simulink model "mars_rover_pose"  (R2023a)
settings: Solver=ode23t  StartTime=0.0  StopTime=2000  FixedStep=1e-2  MaxStep=0.1  RelTol=1e-3  AbsTol=1e-3  EnableMultiTasking=on
StartFcn:
  | mars_rover_sim_callback
model workspace (MATLAB code in the model file):
  | addpath("mars_rover_helpers");
  | % Load Rover Arm model for IK
  | mdlpath = ['mars_rover_data',filesep,'mars_rover_arm'];
  | load_system(mdlpath);
  | 
  | imdata = zeros(3,3,3);
  | 
  | % Temp
  | Kp_steer = 1;
  | Ki_steer = 1;
  | Kd_steer = 1;
  | 
  | Kp = 1;
  | Ki = 1;
  | Kd = 1;
values from neighbouring files (symbols this model uses):
  mapData = false(197,200)    [mars_rover_params.m]    (also in mars_rover_startup.m)
  useKalmanFilter = true    [mars_rover_params.m]
undefined symbols (not defined in the file or in its folder): Arm, armJointAng, armJointTrqs, cameraData, eeConfig, pose, Rover, rover_path_dl, roverPath, sampleLocation, steerAng, steerTrqs, Terrain, vSpeed, Wheel1_G, Wheel2_G, Wheel3_G, Wheel4_G, Wheel5_G, Wheel6_G, wheelTrqs, wSpeeds, X, Y, Z
libraries: sm_lib x238, nesl_utility x80, slpidlib x3, simulink x3, robotcorelib x2, simulink_extras x2, robotalgslib x1
(part 8 of 9)

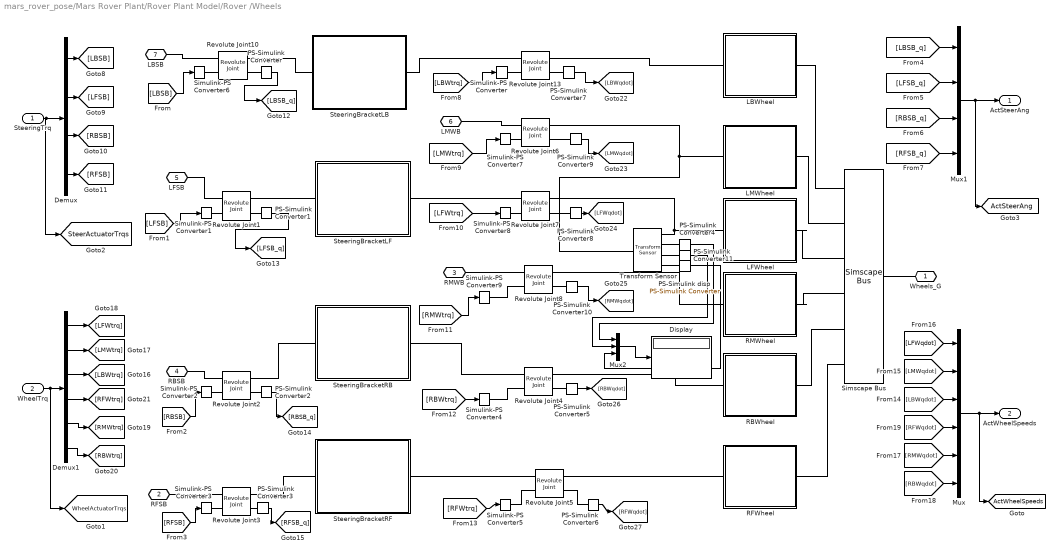
== system mars_rover_pose/Mars Rover Plant/Rover Plant Model/Rover /Wheels ==
  SteeringTrq : Inport
  WheelTrq : Inport  Port=2
  Demux : Demux
  Demux1 : Demux  Outputs=6
  Display : Display
  LBWheel : Subsystem
  LFWheel : Subsystem
  LMWheel : Subsystem
  Mux : Mux  Inputs=6
  Mux1 : Mux
  Mux2 : Mux  Inputs=3
  PS-Simulink Converter{,1..3} (4 alike) : nesl_utility/PS-Simulink Converter  PhysicalDomain=network_engine_domain  SubClassName=ps_output  LeftPortType=input  RightPortType=output  PseudoPeriodic=off  Frequencies=[]  VectorFormat=1-D array  Unit=deg  AffineConversion=off
  PS-Simulink Converter{5..10} (6 alike) : nesl_utility/PS-Simulink Converter  PhysicalDomain=network_engine_domain  SubClassName=ps_output  LeftPortType=input  RightPortType=output  PseudoPeriodic=off  Frequencies=[]  VectorFormat=1-D array  Unit=inherit  AffineConversion=off
  PS-Simulink Converter11 : nesl_utility/PS-Simulink Converter  PhysicalDomain=network_engine_domain  SubClassName=ps_output  LeftPortType=input  RightPortType=output  PseudoPeriodic=off  Frequencies=[]  VectorFormat=inherit  Unit=inherit  AffineConversion=off
  PS-Simulink Converter4 : nesl_utility/PS-Simulink Converter  PhysicalDomain=network_engine_domain  SubClassName=ps_output  LeftPortType=input  RightPortType=output  PseudoPeriodic=off  Frequencies=[]  VectorFormat=inherit  Unit=inherit  AffineConversion=off
  PS-Simulink disp : nesl_utility/PS-Simulink Converter  PhysicalDomain=network_engine_domain  SubClassName=ps_output  LeftPortType=input  RightPortType=output  PseudoPeriodic=off  Frequencies=[]  VectorFormat=inherit  Unit=inherit  AffineConversion=off
  RBWheel : Subsystem
  RFWheel : Subsystem
  RMWheel : Subsystem
  Revolute Joint{1..3,10} (4 alike) : sm_lib/Joints/Revolute Joint  JointMode=Normal  SenseConstraintForce=off  SenseConstraintForceX=off  SenseConstraintForceY=off  SenseConstraintForceZ=off  SenseConstraintTorque=off  SenseConstraintTorqueX=off  SenseConstraintTorqueY=off  SenseConstraintTorqueZ=off  SenseTotalForce=off  SenseTotalForceX=off  SenseTotalForceY=off  SenseTotalForceZ=off  SenseTotalTorque=off  SenseTotalTorqueX=off  SenseTotalTorqueY=off  SenseTotalTorqueZ=off  CompositeWrenchDir=FollowerOnBase  CompositeWrenchFrame=BaseFrame  EquilibriumPosition=0  EquilibriumPositionUnits=deg  SpringStiffness=0  SpringStiffnessUnits=N*m/deg  DampingCoefficient=Rover.steering_damping  DampingCoefficientUnits=N*m/(deg/s)  TorqueActuationMode=InputTorque  MotionActuationMode=ComputedMotion  SensePosition=on  SenseVelocity=off  SenseAcceleration=off  SenseTorqueForce=off  SenseLowerLimitTorqueForce=off  SenseUpperLimitTorqueForce=off  LowerLimitSpecify=off  LowerLimitBound=-90  LowerLimitBoundUnits=deg  LowerLimitStiffness=1e4  LowerLimitStiffnessUnits=N*m/deg  LowerLimitDamping=10  LowerLimitDampingUnits=N*m/(deg/s)  LowerLimitTransitionRegionWidth=0.1  LowerLimitTransitionRegionWidthUnits=deg  UpperLimitSpecify=off  UpperLimitBound=90  UpperLimitBoundUnits=deg  UpperLimitStiffness=1e4  UpperLimitStiffnessUnits=N*m/deg  UpperLimitDamping=10  UpperLimitDampingUnits=N*m/(deg/s)  UpperLimitTransitionRegionWidth=0.1  UpperLimitTransitionRegionWidthUnits=deg  PositionTargetSpecify=on  PositionTargetPriority=High  PositionTargetValue=0  PositionTargetValueUnits=deg  VelocityTargetSpecify=off  VelocityTargetPriority=High  VelocityTargetValue=0  VelocityTargetValueUnits=deg/s
  Revolute Joint{4..8,13} (6 alike) : sm_lib/Joints/Revolute Joint  JointMode=Normal  SenseConstraintForce=off  SenseConstraintForceX=off  SenseConstraintForceY=off  SenseConstraintForceZ=off  SenseConstraintTorque=off  SenseConstraintTorqueX=off  SenseConstraintTorqueY=off  SenseConstraintTorqueZ=off  SenseTotalForce=off  SenseTotalForceX=off  SenseTotalForceY=off  SenseTotalForceZ=off  SenseTotalTorque=off  SenseTotalTorqueX=off  SenseTotalTorqueY=off  SenseTotalTorqueZ=off  CompositeWrenchDir=FollowerOnBase  CompositeWrenchFrame=BaseFrame  EquilibriumPosition=0  EquilibriumPositionUnits=deg  SpringStiffness=0  SpringStiffnessUnits=N*m/deg  DampingCoefficient=Rover.wheel_damping  DampingCoefficientUnits=N*m/(deg/s)  TorqueActuationMode=InputTorque  MotionActuationMode=ComputedMotion  SensePosition=off  SenseVelocity=on  SenseAcceleration=off  SenseTorqueForce=off  SenseLowerLimitTorqueForce=off  SenseUpperLimitTorqueForce=off  LowerLimitSpecify=off  LowerLimitBound=-90  LowerLimitBoundUnits=deg  LowerLimitStiffness=1e4  LowerLimitStiffnessUnits=N*m/deg  LowerLimitDamping=10  LowerLimitDampingUnits=N*m/(deg/s)  LowerLimitTransitionRegionWidth=0.1  LowerLimitTransitionRegionWidthUnits=deg  UpperLimitSpecify=off  UpperLimitBound=90  UpperLimitBoundUnits=deg  UpperLimitStiffness=1e4  UpperLimitStiffnessUnits=N*m/deg  UpperLimitDamping=10  UpperLimitDampingUnits=N*m/(deg/s)  UpperLimitTransitionRegionWidth=0.1  UpperLimitTransitionRegionWidthUnits=deg  PositionTargetSpecify=off  PositionTargetPriority=High  PositionTargetValue=0  PositionTargetValueUnits=deg  VelocityTargetSpecify=off  VelocityTargetPriority=High  VelocityTargetValue=0  VelocityTargetValueUnits=deg/s
  Simscape Bus : SimscapeBus  HierarchyStrings=Wheel1_G;Wheel2_G;Wheel3_G;Wheel4_G;Wheel5_G;Wheel6_G
  Simulink-PS Converter{,4..5,7..9} (6 alike) : nesl_utility/Simulink-PS Converter  PhysicalDomain=network_engine_domain  SubClassName=ps_input  LeftPortType=input  RightPortType=output  PseudoPeriodic=off  Frequencies=[]  NoiseDistribution=none  NoiseParameters=[]  Unit=1  AffineConversion=off  FilteringAndDerivatives=provide  SimscapeFilterOrder=1  InputFilterTimeConstant=0.001  UdotUserProvided=0
  Simulink-PS Converter{1..3,6} (4 alike) : nesl_utility/Simulink-PS Converter  PhysicalDomain=network_engine_domain  SubClassName=ps_input  LeftPortType=input  RightPortType=output  PseudoPeriodic=off  Frequencies=[]  NoiseDistribution=none  NoiseParameters=[]  Unit=1  AffineConversion=off  FilteringAndDerivatives=zero  SimscapeFilterOrder=2  InputFilterTimeConstant=0.001  UdotUserProvided=0
  "SteeringBracketLB " : Subsystem
  SteeringBracketLF : Subsystem
  SteeringBracketRB : Subsystem
  SteeringBracketRF : Subsystem
  Transform Sensor : sm_lib/Frames and Transforms/Transform Sensor  MeasurementFrame=Base  RotationSequence=XYX  SenseAngle=off  SenseAxis=off  SenseQ=off  SenseR=off  SenseRotationSequence=off  SenseOmegaX=off  SenseOmegaY=off  SenseOmegaZ=off  SenseQDot=off  SenseRDot=off  SenseRotationSequenceDot=off  SenseAlphaX=off  SenseAlphaY=off  SenseAlphaZ=off  SenseQDDot=off  SenseRDDot=off  SenseX=on  SenseY=on  SenseZ=on  SenseRad=off  SenseAzim=off  SenseDist=off  SenseInc=off  SenseXDot=off  SenseYDot=off  SenseZDot=off  SenseRadDot=off  SenseAzimDot=off  SenseDistDot=off  SenseIncDot=off  SenseXDDot=off  SenseYDDot=off  SenseZDDot=off  SenseRadDDot=off  SenseAzimDDot=off  SenseDistDDot=off  SenseIncDDot=off
  Wheels_G : PMIOPort  Side=Left
  RFSB : PMIOPort  Port=2  Side=Left
  RMWB : PMIOPort  Port=3  Side=Left
  RBSB : PMIOPort  Port=4  Side=Left
  LFSB : PMIOPort  Port=5  Side=Right
  LMWB : PMIOPort  Port=6  Side=Right
  LBSB : PMIOPort  Port=7  Side=Right
  ActSteerAng : Outport
  ActWheelSpeeds : Outport  Port=2
  tag scope: ActSteerAng=global, ActWheelSpeeds=global, SteerActuatorTrqs=global, WheelActuatorTrqs=global
  wires:
  SteeringTrq/1 -> [SteerActuatorTrqs], Demux/1
  Mux1/1 -> ActSteerAng/1, [ActSteerAng]
  WheelTrq/1 -> Demux1/1, [WheelActuatorTrqs]
  [LBSB] -> Simulink-PS Converter6/1
  Demux/1 -> [LBSB]
  Demux/2 -> [LFSB]
  Demux/3 -> [RBSB]
  Demux/4 -> [RFSB]
  [LFSB] -> Simulink-PS Converter1/1
  [RBSB] -> Simulink-PS Converter2/1
  [RFSB] -> Simulink-PS Converter3/1
  [LBSB_q] -> Mux1/1
  [LFSB_q] -> Mux1/2
  [RBSB_q] -> Mux1/3
  [RFSB_q] -> Mux1/4
  PS-Simulink Converter/1 -> [LBSB_q]
  PS-Simulink Converter1/1 -> [LFSB_q]
  PS-Simulink Converter2/1 -> [RBSB_q]
  PS-Simulink Converter3/1 -> [RFSB_q]
  [LBWtrq] -> Simulink-PS Converter/1
  [LMWtrq] -> Simulink-PS Converter7/1
  Demux1/3 -> [LBWtrq]
  Demux1/2 -> [LMWtrq]
  [LFWtrq] -> Simulink-PS Converter8/1
  Demux1/1 -> [LFWtrq]
  [RMWtrq] -> Simulink-PS Converter9/1
  Demux1/5 -> [RMWtrq]
  [RBWtrq] -> Simulink-PS Converter4/1
  Demux1/6 -> [RBWtrq]
  [RFWtrq] -> Simulink-PS Converter5/1
  Demux1/4 -> [RFWtrq]
  PS-Simulink Converter7/1 -> [LBWqdot]
  [LBWqdot] -> Mux/3
  PS-Simulink Converter9/1 -> [LMWqdot]
  [LMWqdot] -> Mux/2
  PS-Simulink Converter8/1 -> [LFWqdot]
  [LFWqdot] -> Mux/1
  PS-Simulink Converter10/1 -> [RMWqdot]
  PS-Simulink Converter5/1 -> [RBWqdot]
  PS-Simulink Converter6/1 -> [RFWqdot]
  [RMWqdot] -> Mux/5
  [RBWqdot] -> Mux/6
  [RFWqdot] -> Mux/4
  Mux/1 -> ActWheelSpeeds/1, [ActWheelSpeeds]
  Mux2/1 -> Display/1
  PS-Simulink Converter4/1 -> Mux2/1
  PS-Simulink Converter11/1 -> Mux2/2
  PS-Simulink disp/1 -> Mux2/3
  connections:
  PS-Simulink Converter/LConn1 -- Revolute Joint10/RConn2
  Revolute Joint10/LConn1 -- LBSB/RConn1
  Simulink-PS Converter6/RConn1 -- Revolute Joint10/LConn2
  "SteeringBracketLB "/LConn1 -- Revolute Joint10/RConn1
  Revolute Joint6/LConn1 -- LMWB/RConn1
  LFSB/RConn1 -- Revolute Joint1/LConn1
  Revolute Joint8/LConn1 -- RMWB/RConn1
  RBSB/RConn1 -- Revolute Joint2/LConn1
  PS-Simulink Converter1/LConn1 -- Revolute Joint1/RConn2
  Simulink-PS Converter1/RConn1 -- Revolute Joint1/LConn2
  Revolute Joint2/RConn1 -- SteeringBracketRB/LConn1
  PS-Simulink Converter2/LConn1 -- Revolute Joint2/RConn2
  Simulink-PS Converter2/RConn1 -- Revolute Joint2/LConn2
  RFSB/RConn1 -- Revolute Joint3/LConn1
  Revolute Joint3/RConn1 -- SteeringBracketRF/LConn1
  Simulink-PS Converter3/RConn1 -- Revolute Joint3/LConn2
  PS-Simulink Converter3/LConn1 -- Revolute Joint3/RConn2
  Wheels_G/RConn1 -- Simscape Bus/RConn1
  LMWheel/LConn1 -- Simscape Bus/LConn2
  RMWheel/LConn1 -- Simscape Bus/LConn4
  LFWheel/LConn1 -- Simscape Bus/LConn3
  Revolute Joint4/LConn1 -- SteeringBracketRB/RConn1
  Revolute Joint1/RConn1 -- SteeringBracketLF/LConn1
  Revolute Joint4/RConn1 -- RBWheel/RConn1
  LBWheel/RConn1 -- Revolute Joint13/RConn1
  LMWheel/RConn1 -- Revolute Joint6/RConn1 -- Transform Sensor/LConn1
  PS-Simulink Converter6/LConn1 -- Revolute Joint5/RConn2
  Revolute Joint8/LConn2 -- Simulink-PS Converter9/RConn1
  Revolute Joint13/LConn1 -- "SteeringBracketLB "/RConn1
  Simscape Bus/LConn5 -- RBWheel/LConn1
  Simulink-PS Converter5/RConn1 -- Revolute Joint5/LConn2
  Revolute Joint4/RConn2 -- PS-Simulink Converter5/LConn1
  Revolute Joint8/RConn2 -- PS-Simulink Converter10/LConn1
  Revolute Joint4/LConn2 -- Simulink-PS Converter4/RConn1
  Revolute Joint5/LConn1 -- SteeringBracketRF/RConn1
  Revolute Joint6/LConn2 -- Simulink-PS Converter7/RConn1
  Revolute Joint6/RConn2 -- PS-Simulink Converter9/LConn1
  Simscape Bus/LConn1 -- LBWheel/LConn1
  Revolute Joint13/RConn2 -- PS-Simulink Converter7/LConn1
  Revolute Joint7/LConn2 -- Simulink-PS Converter8/RConn1
  Revolute Joint7/RConn2 -- PS-Simulink Converter8/LConn1
  RMWheel/RConn1 -- Revolute Joint8/RConn1
  Revolute Joint7/LConn1 -- SteeringBracketLF/RConn1
  Simulink-PS Converter/RConn1 -- Revolute Joint13/LConn2
  LFWheel/RConn1 -- Revolute Joint7/RConn1 -- Transform Sensor/RConn1
  RFWheel/LConn1 -- Simscape Bus/LConn6
  Revolute Joint5/RConn1 -- RFWheel/RConn1
  PS-Simulink Converter4/LConn1 -- Transform Sensor/RConn2
  PS-Simulink Converter11/LConn1 -- Transform Sensor/RConn3
  PS-Simulink disp/LConn1 -- Transform Sensor/RConn4

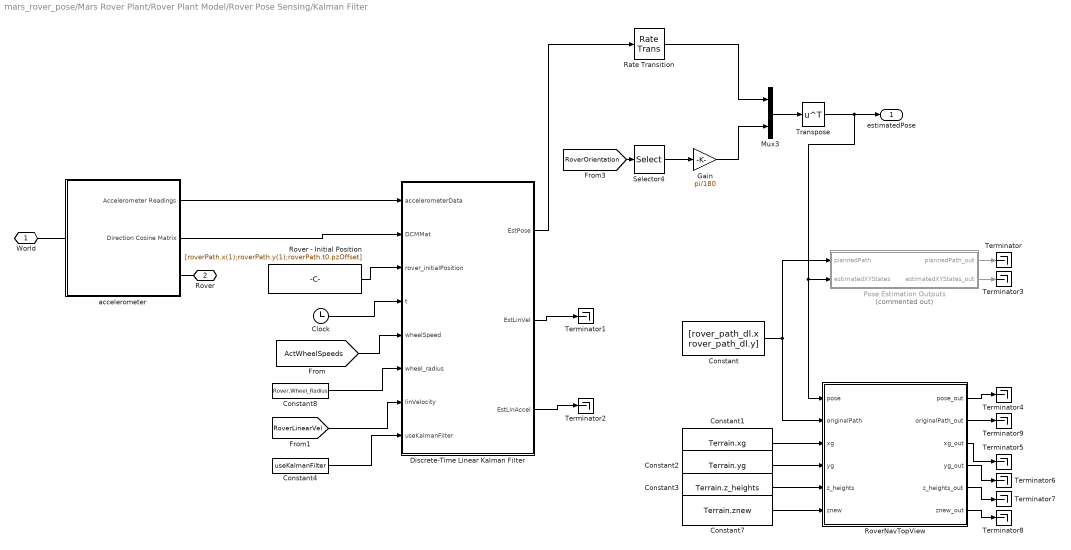
== system mars_rover_pose/Mars Rover Plant/Rover Plant Model/Rover Pose Sensing/Kalman Filter ==
  Clock : Clock
  Constant : Constant  Value=[rover_path_dl.x rover_path_dl.y]
  Constant1 : Constant  Value=Terrain.xg
  Constant2 : Constant  Value=Terrain.yg
  Constant3 : Constant  Value=Terrain.z_heights
  Constant4 : Constant  Value=useKalmanFilter
  Constant7 : Constant  Value=Terrain.znew
  Constant8 : Constant  Value=Rover.Wheel_Radius
  Discrete-Time Linear Kalman Filter : MATLAB Function  TreatAsAtomicUnit=on
  Gain : Gain  Gain=pi/180
  Mux3 : Mux  Inputs=2
  Pose Estimation Outputs : MATLAB Function  Commented=on  TreatAsAtomicUnit=on
  Rate Transition : RateTransition  InitialCondition=[roverPath.x(1) roverPath.y(1)]  OutPortSampleTime=10
  Rover - Initial Position : Constant  Value=[roverPath.x(1);roverPath.y(1);roverPath.t0.pzOffset]
  RoverNavTopView : MATLAB Function  TreatAsAtomicUnit=on
  Selector4 : Selector  InputPortWidth=3  IndexOptions=Index vector (dialog)  Indices=3  OutputSizes=1
  Terminator{,1..9} (10 alike) : Terminator
  Transpose : Math  Operator=transpose
  accelerometer : Subsystem
  World : PMIOPort  Side=Left
  Rover : PMIOPort  Port=2  Side=Right
  estimatedPose : Outport
  wires:
  Discrete-Time Linear Kalman Filter/2(EstLinVel) -> Terminator1/1
  Selector4/1 -> Gain/1
  accelerometer/2(Direction Cosine Matrix) -> Discrete-Time Linear Kalman Filter/2(DCMMat)
  [RoverOrientation] -> Selector4/1
  Discrete-Time Linear Kalman Filter/3(EstLinAccel) -> Terminator2/1
  accelerometer/1(Accelerometer Readings) -> Discrete-Time Linear Kalman Filter/1(accelerometerData)
  Constant8/1 -> Discrete-Time Linear Kalman Filter/6(wheel_radius)
  Rover - Initial Position/1 -> Discrete-Time Linear Kalman Filter/3(rover_initialPosition)
  Transpose/1 -> RoverNavTopView/1(pose), Pose Estimation Outputs/2(estimatedXYStates), estimatedPose/1
  Discrete-Time Linear Kalman Filter/1(EstPose) -> Rate Transition/1
  Mux3/1 -> Transpose/1
  Gain/1 -> Mux3/2
  Rate Transition/1 -> Mux3/1
  [ActWheelSpeeds] -> Discrete-Time Linear Kalman Filter/5(wheelSpeed)
  Clock/1 -> Discrete-Time Linear Kalman Filter/4(t)
  [RoverLinearVel] -> Discrete-Time Linear Kalman Filter/7(linVelocity)
  Pose Estimation Outputs/1(plannedPath_out) -> Terminator/1
  Pose Estimation Outputs/2(estimatedXYStates_out) -> Terminator3/1
  Constant/1 -> RoverNavTopView/2(originalPath), Pose Estimation Outputs/1(plannedPath)
  Constant3/1 -> RoverNavTopView/5(z_heights)
  Constant2/1 -> RoverNavTopView/4(yg)
  Constant1/1 -> RoverNavTopView/3(xg)
  RoverNavTopView/3(xg_out) -> Terminator5/1
  Constant7/1 -> RoverNavTopView/6(znew)
  RoverNavTopView/5(z_heights_out) -> Terminator7/1
  RoverNavTopView/4(yg_out) -> Terminator6/1
  RoverNavTopView/6(znew_out) -> Terminator8/1
  RoverNavTopView/1(pose_out) -> Terminator4/1
  RoverNavTopView/2(originalPath_out) -> Terminator9/1
  Constant4/1 -> Discrete-Time Linear Kalman Filter/8(useKalmanFilter)
  connections:
  accelerometer/LConn1 -- World/RConn1
  accelerometer/RConn1 -- Rover/RConn1

== system mars_rover_pose/Mars Rover Plant/Rover Plant Model/Rover Pose Sensing/Subsystem ==
  posX : Inport
  vx : Inport  Port=2
  posY : Inport  Port=3
  vy : Inport  Port=4
  posZ : Inport  Port=5
  Q : Inport  Port=6
  CalcSpeed : MATLAB Function  TreatAsAtomicUnit=on
  Mux : Mux  Inputs=3
  Mux1 : Mux  Inputs=2
  Mux2 : Mux  Inputs=3
  Mux3 : Mux  Inputs=3
  Radians to Degrees : simulink_extras/Transformations/Radians to Degrees
  theta_act : MATLAB Function  TreatAsAtomicUnit=on
  pose : Outport
  xyz : Outport  Port=2
  linVelxy : Outport  Port=3
  vSpeed : Outport  Port=4
  rotang : Outport  Port=5
  wires:
  posY/1 -> Mux/2, Mux3/2
  Mux1/1 -> linVelxy/1, CalcSpeed/1(u)
  Mux2/1 -> Radians to Degrees/1
  theta_act/1(z) -> Mux2/3, Mux/3
  Radians to Degrees/1 -> rotang/1
  theta_act/3(x) -> Mux2/1
  theta_act/2(y) -> Mux2/2
  posX/1 -> Mux3/1, Mux/1
  vx/1 -> Mux1/1
  Mux/1 -> pose/1
  Q/1 -> theta_act/1(u)
  vy/1 -> Mux1/2
  posZ/1 -> Mux3/3
  CalcSpeed/1(y) -> vSpeed/1
  Mux3/1 -> xyz/1

== system mars_rover_pose/Perception/sceneViewer/Stereo_Left/drawScene ==
  Camera_Z_ang : Inport
  Camera_pos : Inport  Port=2
  Camera_rot : Inport  Port=3
  Camera_target_ang : Inport  Port=4
  xg : Inport  Port=5
  yg : Inport  Port=6
  z_heights : Inport  Port=7
  znew : Inport  Port=8
  rover_path_x : Inport  Port=9
  rover_path_y : Inport  Port=10
  rover_path_z : Inport  Port=11
  Trigger : TriggerPort  VariantControl=(inherit)  InitialTriggerSignalState=negative  PortDimensions=1
  Camera : MATLAB Function  TreatAsAtomicUnit=on
  im : Outport
  wires:
  Camera/1(im) -> im/1
  rover_path_x/1 -> Camera/9(rover_path_x)
  Camera_Z_ang/1 -> Camera/1(Camera_Z_ang)
  rover_path_z/1 -> Camera/11(rover_path_z)
  z_heights/1 -> Camera/7(z_heights)
  xg/1 -> Camera/5(xg)
  znew/1 -> Camera/8(znew)
  rover_path_y/1 -> Camera/10(rover_path_y)
  yg/1 -> Camera/6(yg)
  Camera_pos/1 -> Camera/2(Camera_pos)
  Camera_target_ang/1 -> Camera/4(Camera_target_ang)
  Camera_rot/1 -> Camera/3(Camera_rot)

== system mars_rover_pose/Perception/sceneViewer/Stereo_Right/drawScene ==
  Camera_Z_ang : Inport
  Camera_pos : Inport  Port=2
  Camera_rot : Inport  Port=3
  Camera_target_ang : Inport  Port=4
  xg : Inport  Port=5
  yg : Inport  Port=6
  z_heights : Inport  Port=7
  znew : Inport  Port=8
  rover_path_x : Inport  Port=9
  rover_path_y : Inport  Port=10
  rover_path_z : Inport  Port=11
  Trigger : TriggerPort  VariantControl=(inherit)  InitialTriggerSignalState=negative  PortDimensions=1
  Camera : MATLAB Function  TreatAsAtomicUnit=on
  im : Outport
  wires:
  Camera/1(im) -> im/1
  Camera_pos/1 -> Camera/2(Camera_pos)
  rover_path_z/1 -> Camera/11(rover_path_z)
  Camera_target_ang/1 -> Camera/4(Camera_target_ang)
  rover_path_y/1 -> Camera/10(rover_path_y)
  znew/1 -> Camera/8(znew)
  z_heights/1 -> Camera/7(z_heights)
  xg/1 -> Camera/5(xg)
  rover_path_x/1 -> Camera/9(rover_path_x)
  yg/1 -> Camera/6(yg)
  Camera_Z_ang/1 -> Camera/1(Camera_Z_ang)
  Camera_rot/1 -> Camera/3(Camera_rot)

== system mars_rover_pose/Control/Manipulator Control/ Trajectory Planner/SampleDropOffCmdLogic/Enabled Subsystem1 ==
  In1 : Inport
  Enable : EnablePort
  Out1 : Outport
  wires:
  In1/1 -> Out1/1

== system mars_rover_pose/Control/Manipulator Control/ Trajectory Planner/SampleLoc wrt arm base/Enabled Subsystem1 ==
  In1 : Inport
  Enable : EnablePort
  Out1 : Outport
  wires:
  In1/1 -> Out1/1

== system mars_rover_pose/Control/Manipulator Control/ Trajectory Planner/SamplePickUpCmdLogic/Enabled Subsystem1 ==
  In1 : Inport
  Enable : EnablePort
  Out1 : Outport
  wires:
  In1/1 -> Out1/1

== system mars_rover_pose/Control/Rover Control/Rover Path Planning And Control/Ackerman Steer Angle/Enabled Subsystem ==
  In1 : Inport
  Enable : EnablePort
  delta : Outport
  wires:
  In1/1 -> delta/1

== system mars_rover_pose/Control/Rover Control/Rover Path Planning And Control/hold/RoverStopTime ==
  Enable : Inport
  Clock : Clock
  Constant2 : Constant
  Display : Display
  Enabled Subsystem1 : Subsystem  TreatAsAtomicUnit=on
      settings: MinAlgLoopOccurrences=on
  Switch : Switch  Criteria=u2 > Threshold  SaturateOnIntegerOverflow=off  InputSameDT=off
  Unit Delay : UnitDelay  SampleTime=-1  HasFrameUpgradeWarning=on
  DeAccelTime : Outport
  wires:
  Enabled Subsystem1/1(Out1) -> Switch/2
  Enable/1 -> Enabled Subsystem1/Enable
  Switch/1 -> Unit Delay/1
  Unit Delay/1 -> Display/1, DeAccelTime/1, Switch/1
  Clock/1 -> Switch/3
  Constant2/1 -> Enabled Subsystem1/1(In1)

== system mars_rover_pose/Mars Rover Plant/Manipulator Plant Model/SampleGeneration/SampleLoc wrt arm base/Enabled Subsystem1 ==
  In1 : Inport
  Enable : EnablePort
  Out1 : Outport
  wires:
  In1/1 -> Out1/1

== system mars_rover_pose/Mars Rover Plant/Rover Plant Model/Rover /Wheels/LBWheel ==
  InnerWheelViz : sm_lib/Body Elements/File Solid  ExtGeomFileName=mobility_wheel_inner.stl  UnitType=Custom  ExtGeomFileUnits=cm  StepReaderType=HEX  ExportConvexHullGeometry=off  InertiaType=Custom  Mass=0  MassUnits=kg  CenterOfMass=[0 0 0]  CenterOfMassUnits=m  MomentsOfInertia=[1 1 1]*0  MomentsOfInertiaUnits=kg*m^2  ProductsOfInertia=[0 0 0]  ProductsOfInertiaUnits=kg*m^2  BasedOnType=Density  Density=1000  DensityUnits=kg/m^3  DoExposeReferenceFrame=on  SerializedFrames=<Frames/>  GraphicType=FromGeometry  MarkerShape=Sphere  MarkerSize=10  GraphicVisPropType=AdvancedVisualProperties  GraphicDiffuseColor=[1.0 1.0 1.0]  GraphicSpecularColor=[1 1 1 1.0]  GraphicAmbientColor=[0.15 0.15 0.15 1.0]  GraphicEmissiveColor=[0.1 0.1 0 1.0]  GraphicShininess=90  GraphicOpacity=1.0
  OuterWheel : sm_lib/Body Elements/File Solid  ExtGeomFileName=mobility_wheel_outer.stl  UnitType=Custom  ExtGeomFileUnits=cm  StepReaderType=HEX  ExportConvexHullGeometry=off  InertiaType=CalculateFromGeometry  Mass=1  MassUnits=kg  CenterOfMass=[0 0 0]  CenterOfMassUnits=m  MomentsOfInertia=[1 1 1]  MomentsOfInertiaUnits=kg*m^2  ProductsOfInertia=[0 0 0]  ProductsOfInertiaUnits=kg*m^2  BasedOnType=Density  Density=2700  DensityUnits=kg/m^3  DoExposeReferenceFrame=on  SerializedFrames=<Frames/>  GraphicType=FromGeometry  MarkerShape=Sphere  MarkerSize=10  GraphicVisPropType=AdvancedVisualProperties  GraphicDiffuseColor=[0.15 0.15 0.15]  GraphicSpecularColor=[1 1 1 1.0]  GraphicAmbientColor=[0.15 0.15 0.15 1.0]  GraphicEmissiveColor=[0. 0. 0. 1]  GraphicShininess=100  GraphicOpacity=1.0
  Point Cloud : sm_lib/Curves and Surfaces/Point Cloud  CoordinatesMatrix=Rover.new_wheel_points  CoordinatesMatrixUnits=cm  GraphicType=MarkerCloud  GraphicSphereRadius=0.5  GraphicSphereRadiusUnits=cm  GraphicVisPropType=SimpleVisualProperties  GraphicDiffuseColor=[0.07451 0.6235 1]  GraphicOpacity=1.0  GraphicSpecularColor=[0.5 0.5 0.5 1.0]  GraphicAmbientColor=[0.15 0.15 0.15 1.0]  GraphicEmissiveColor=[0.0 0.0 0.0 1.0]  GraphicShininess=75
  Rigid Transform : sm_lib/Frames and Transforms/Rigid Transform  TranslationMethod=Cartesian  TranslationStandardOffset=0  TranslationStandardOffsetUnits=m  TranslationStandardAxis=+Z  TranslationCartesianOffset=Rover.Wheel.WRJ_T  TranslationCartesianOffsetUnits=m  TranslationROffset=0  TranslationROffsetUnits=m  TranslationZOffset=0  TranslationZOffsetUnits=m  TranslationThetaOffset=0  TranslationThetaOffsetUnits=deg  RotationMethod=RotationMatrix  RotationAngleUnits=deg  RotationStandardAxis=+Z  RotationAngle=0.0  RotationArbitraryAxis=[0 0 1]  FollAlignAxisA=+X  BaseAlignAxisA=+Y  FollAlignAxisB=+Y  BaseAlignAxisB=+Z  RotationSequenceAxes=FollowerAxes  RotationSequence=XYX  RotationSequenceAngles=[0 0 0]  RotationSequenceAnglesUnits=deg  RotationMatrix=Rover.Wheel.WRJ_R  Quaternion=[1 0 0 0]
  Rigid Transform6 : sm_lib/Frames and Transforms/Rigid Transform  TranslationMethod=StandardAxis  TranslationStandardOffset=25.500/2  TranslationStandardOffsetUnits=cm  TranslationStandardAxis=+Y  TranslationCartesianOffset=[0 0 0]  TranslationCartesianOffsetUnits=cm  TranslationROffset=0  TranslationROffsetUnits=m  TranslationZOffset=0  TranslationZOffsetUnits=m  TranslationThetaOffset=0  TranslationThetaOffsetUnits=deg  RotationMethod=StandardAxis  RotationAngleUnits=deg  RotationStandardAxis=+X  RotationAngle=90  RotationArbitraryAxis=[0 0 1]  FollAlignAxisA=+X  BaseAlignAxisA=+Y  FollAlignAxisB=+Y  BaseAlignAxisB=+Z  RotationSequenceAxes=FollowerAxes  RotationSequence=XYX  RotationSequenceAngles=[0 0 0]  RotationSequenceAnglesUnits=deg  RotationMatrix=[1 0 0; 0 1 0; 0 0 1]  Quaternion=[1 0 0 0]
  WRJ : PMIOPort  Side=Right
  G : PMIOPort  Port=2  Side=Left
  connections:
  Rigid Transform6/RConn1 -- Rigid Transform/RConn1 -- WRJ/RConn1
  OuterWheel/RConn1 -- Point Cloud/LConn1 -- Rigid Transform6/LConn1
  G/RConn1 -- Point Cloud/RConn1
  InnerWheelViz/RConn1 -- Rigid Transform/LConn1

== system mars_rover_pose/Mars Rover Plant/Rover Plant Model/Rover /Wheels/LFWheel ==
  InnerWheel : sm_lib/Body Elements/File Solid  ExtGeomFileName=mobility_wheel_inner.stl  UnitType=Custom  ExtGeomFileUnits=cm  StepReaderType=HEX  ExportConvexHullGeometry=off  InertiaType=Custom  Mass=0  MassUnits=kg  CenterOfMass=[0 0 0]  CenterOfMassUnits=m  MomentsOfInertia=[1 1 1]*0  MomentsOfInertiaUnits=kg*m^2  ProductsOfInertia=[0 0 0]  ProductsOfInertiaUnits=kg*m^2  BasedOnType=Density  Density=1000  DensityUnits=kg/m^3  DoExposeReferenceFrame=on  SerializedFrames=<Frames/>  GraphicType=FromGeometry  MarkerShape=Sphere  MarkerSize=10  GraphicVisPropType=AdvancedVisualProperties  GraphicDiffuseColor=[1.0 1.0 1.0]  GraphicSpecularColor=[1 1 1 1.0]  GraphicAmbientColor=[0.15 0.15 0.15 1.0]  GraphicEmissiveColor=[0.1 0.1 0 1.0]  GraphicShininess=90  GraphicOpacity=1.0
  OuterWheel : sm_lib/Body Elements/File Solid  ExtGeomFileName=mobility_wheel_outer.stl  UnitType=Custom  ExtGeomFileUnits=cm  StepReaderType=HEX  ExportConvexHullGeometry=off  InertiaType=CalculateFromGeometry  Mass=1  MassUnits=kg  CenterOfMass=[0 0 0]  CenterOfMassUnits=m  MomentsOfInertia=[1 1 1]  MomentsOfInertiaUnits=kg*m^2  ProductsOfInertia=[0 0 0]  ProductsOfInertiaUnits=kg*m^2  BasedOnType=Density  Density=2700  DensityUnits=kg/m^3  DoExposeReferenceFrame=on  SerializedFrames=<Frames/>  GraphicType=FromGeometry  MarkerShape=Sphere  MarkerSize=10  GraphicVisPropType=AdvancedVisualProperties  GraphicDiffuseColor=[0.15 0.15 0.15]  GraphicSpecularColor=[1 1 1 1.0]  GraphicAmbientColor=[0.15 0.15 0.15 1.0]  GraphicEmissiveColor=[0. 0. 0. 1]  GraphicShininess=100  GraphicOpacity=1.0
  Point Cloud : sm_lib/Curves and Surfaces/Point Cloud  CoordinatesMatrix=Rover.new_wheel_points  CoordinatesMatrixUnits=cm  GraphicType=MarkerCloud  GraphicSphereRadius=0.5  GraphicSphereRadiusUnits=cm  GraphicVisPropType=SimpleVisualProperties  GraphicDiffuseColor=[0.07451 0.6235 1]  GraphicOpacity=1.0  GraphicSpecularColor=[0.5 0.5 0.5 1.0]  GraphicAmbientColor=[0.15 0.15 0.15 1.0]  GraphicEmissiveColor=[0.0 0.0 0.0 1.0]  GraphicShininess=75
  Rigid Transform : sm_lib/Frames and Transforms/Rigid Transform  TranslationMethod=Cartesian  TranslationStandardOffset=0  TranslationStandardOffsetUnits=m  TranslationStandardAxis=+Z  TranslationCartesianOffset=Rover.Wheel.WRJ_T  TranslationCartesianOffsetUnits=m  TranslationROffset=0  TranslationROffsetUnits=m  TranslationZOffset=0  TranslationZOffsetUnits=m  TranslationThetaOffset=0  TranslationThetaOffsetUnits=deg  RotationMethod=RotationMatrix  RotationAngleUnits=deg  RotationStandardAxis=+Z  RotationAngle=0.0  RotationArbitraryAxis=[0 0 1]  FollAlignAxisA=+X  BaseAlignAxisA=+Y  FollAlignAxisB=+Y  BaseAlignAxisB=+Z  RotationSequenceAxes=FollowerAxes  RotationSequence=XYX  RotationSequenceAngles=[0 0 0]  RotationSequenceAnglesUnits=deg  RotationMatrix=Rover.Wheel.WRJ_R  Quaternion=[1 0 0 0]
  Rigid Transform6 : sm_lib/Frames and Transforms/Rigid Transform  TranslationMethod=StandardAxis  TranslationStandardOffset=25.500/2  TranslationStandardOffsetUnits=cm  TranslationStandardAxis=+Y  TranslationCartesianOffset=[0 0 0]  TranslationCartesianOffsetUnits=cm  TranslationROffset=0  TranslationROffsetUnits=m  TranslationZOffset=0  TranslationZOffsetUnits=m  TranslationThetaOffset=0  TranslationThetaOffsetUnits=deg  RotationMethod=StandardAxis  RotationAngleUnits=deg  RotationStandardAxis=+X  RotationAngle=90  RotationArbitraryAxis=[0 0 1]  FollAlignAxisA=+X  BaseAlignAxisA=+Y  FollAlignAxisB=+Y  BaseAlignAxisB=+Z  RotationSequenceAxes=FollowerAxes  RotationSequence=XYX  RotationSequenceAngles=[0 0 0]  RotationSequenceAnglesUnits=deg  RotationMatrix=[1 0 0; 0 1 0; 0 0 1]  Quaternion=[1 0 0 0]
  WRJ : PMIOPort  Side=Right
  G : PMIOPort  Port=2  Side=Left
  connections:
  Rigid Transform6/RConn1 -- WRJ/RConn1 -- Rigid Transform/RConn1
  OuterWheel/RConn1 -- Point Cloud/LConn1 -- Rigid Transform6/LConn1
  G/RConn1 -- Point Cloud/RConn1
  InnerWheel/RConn1 -- Rigid Transform/LConn1

== system mars_rover_pose/Mars Rover Plant/Rover Plant Model/Rover /Wheels/LMWheel ==
  InnerWheel : sm_lib/Body Elements/File Solid  ExtGeomFileName=mobility_wheel_inner.stl  UnitType=Custom  ExtGeomFileUnits=cm  StepReaderType=HEX  ExportConvexHullGeometry=off  InertiaType=Custom  Mass=0  MassUnits=kg  CenterOfMass=[0 0 0]  CenterOfMassUnits=m  MomentsOfInertia=[1 1 1]*0  MomentsOfInertiaUnits=kg*m^2  ProductsOfInertia=[0 0 0]  ProductsOfInertiaUnits=kg*m^2  BasedOnType=Density  Density=1000  DensityUnits=kg/m^3  DoExposeReferenceFrame=on  SerializedFrames=<Frames/>  GraphicType=FromGeometry  MarkerShape=Sphere  MarkerSize=10  GraphicVisPropType=AdvancedVisualProperties  GraphicDiffuseColor=[1.0 1.0 1.0]  GraphicSpecularColor=[1 1 1 1.0]  GraphicAmbientColor=[0.15 0.15 0.15 1.0]  GraphicEmissiveColor=[0.1 0.1 0 1.0]  GraphicShininess=90  GraphicOpacity=1.0
  OuterWheel : sm_lib/Body Elements/File Solid  ExtGeomFileName=mobility_wheel_outer.stl  UnitType=Custom  ExtGeomFileUnits=cm  StepReaderType=HEX  ExportConvexHullGeometry=off  InertiaType=CalculateFromGeometry  Mass=1  MassUnits=kg  CenterOfMass=[0 0 0]  CenterOfMassUnits=m  MomentsOfInertia=[1 1 1]  MomentsOfInertiaUnits=kg*m^2  ProductsOfInertia=[0 0 0]  ProductsOfInertiaUnits=kg*m^2  BasedOnType=Density  Density=2700  DensityUnits=kg/m^3  DoExposeReferenceFrame=on  SerializedFrames=<Frames/>  GraphicType=FromGeometry  MarkerShape=Sphere  MarkerSize=10  GraphicVisPropType=AdvancedVisualProperties  GraphicDiffuseColor=[0.15 0.15 0.15]  GraphicSpecularColor=[1 1 1 1.0]  GraphicAmbientColor=[0.15 0.15 0.15 1.0]  GraphicEmissiveColor=[0. 0. 0. 1]  GraphicShininess=100  GraphicOpacity=1.0
  Point Cloud : sm_lib/Curves and Surfaces/Point Cloud  CoordinatesMatrix=Rover.new_wheel_points  CoordinatesMatrixUnits=cm  GraphicType=MarkerCloud  GraphicSphereRadius=0.5  GraphicSphereRadiusUnits=cm  GraphicVisPropType=SimpleVisualProperties  GraphicDiffuseColor=[0.07451 0.6235 1]  GraphicOpacity=1.0  GraphicSpecularColor=[0.5 0.5 0.5 1.0]  GraphicAmbientColor=[0.15 0.15 0.15 1.0]  GraphicEmissiveColor=[0.0 0.0 0.0 1.0]  GraphicShininess=75
  Rigid Transform : sm_lib/Frames and Transforms/Rigid Transform  TranslationMethod=Cartesian  TranslationStandardOffset=0  TranslationStandardOffsetUnits=m  TranslationStandardAxis=+Z  TranslationCartesianOffset=Rover.Wheel.WRJ_T  TranslationCartesianOffsetUnits=m  TranslationROffset=0  TranslationROffsetUnits=m  TranslationZOffset=0  TranslationZOffsetUnits=m  TranslationThetaOffset=0  TranslationThetaOffsetUnits=deg  RotationMethod=RotationMatrix  RotationAngleUnits=deg  RotationStandardAxis=+Z  RotationAngle=0.0  RotationArbitraryAxis=[0 0 1]  FollAlignAxisA=+X  BaseAlignAxisA=+Y  FollAlignAxisB=+Y  BaseAlignAxisB=+Z  RotationSequenceAxes=FollowerAxes  RotationSequence=XYX  RotationSequenceAngles=[0 0 0]  RotationSequenceAnglesUnits=deg  RotationMatrix=Rover.Wheel.WRJ_R  Quaternion=[1 0 0 0]
  Rigid Transform6 : sm_lib/Frames and Transforms/Rigid Transform  TranslationMethod=StandardAxis  TranslationStandardOffset=25.500/2  TranslationStandardOffsetUnits=cm  TranslationStandardAxis=+Y  TranslationCartesianOffset=[0 0 0]  TranslationCartesianOffsetUnits=cm  TranslationROffset=0  TranslationROffsetUnits=m  TranslationZOffset=0  TranslationZOffsetUnits=m  TranslationThetaOffset=0  TranslationThetaOffsetUnits=deg  RotationMethod=StandardAxis  RotationAngleUnits=deg  RotationStandardAxis=+X  RotationAngle=90  RotationArbitraryAxis=[0 0 1]  FollAlignAxisA=+X  BaseAlignAxisA=+Y  FollAlignAxisB=+Y  BaseAlignAxisB=+Z  RotationSequenceAxes=FollowerAxes  RotationSequence=XYX  RotationSequenceAngles=[0 0 0]  RotationSequenceAnglesUnits=deg  RotationMatrix=[1 0 0; 0 1 0; 0 0 1]  Quaternion=[1 0 0 0]
  WRJ : PMIOPort  Side=Right
  G : PMIOPort  Port=2  Side=Left
  connections:
  InnerWheel/RConn1 -- Rigid Transform/LConn1
  G/RConn1 -- Point Cloud/RConn1
  Rigid Transform6/LConn1 -- Point Cloud/LConn1 -- OuterWheel/RConn1
  Rigid Transform/RConn1 -- WRJ/RConn1 -- Rigid Transform6/RConn1

== system mars_rover_pose/Mars Rover Plant/Rover Plant Model/Rover /Wheels/RBWheel ==
  InnerWheel : sm_lib/Body Elements/File Solid  ExtGeomFileName=mobility_wheel_inner.stl  UnitType=Custom  ExtGeomFileUnits=cm  StepReaderType=HEX  ExportConvexHullGeometry=off  InertiaType=Custom  Mass=0  MassUnits=kg  CenterOfMass=[0 0 0]  CenterOfMassUnits=m  MomentsOfInertia=[1 1 1]*0  MomentsOfInertiaUnits=kg*m^2  ProductsOfInertia=[0 0 0]  ProductsOfInertiaUnits=kg*m^2  BasedOnType=Density  Density=1000  DensityUnits=kg/m^3  DoExposeReferenceFrame=on  SerializedFrames=<Frames/>  GraphicType=FromGeometry  MarkerShape=Sphere  MarkerSize=10  GraphicVisPropType=AdvancedVisualProperties  GraphicDiffuseColor=[1.0 1.0 1.0]  GraphicSpecularColor=[1 1 1 1.0]  GraphicAmbientColor=[0.15 0.15 0.15 1.0]  GraphicEmissiveColor=[0.1 0.1 0 1.0]  GraphicShininess=90  GraphicOpacity=1.0
  OuterWheel : sm_lib/Body Elements/File Solid  ExtGeomFileName=mobility_wheel_outer.stl  UnitType=Custom  ExtGeomFileUnits=cm  StepReaderType=HEX  ExportConvexHullGeometry=off  InertiaType=CalculateFromGeometry  Mass=1  MassUnits=kg  CenterOfMass=[0 0 0]  CenterOfMassUnits=m  MomentsOfInertia=[1 1 1]  MomentsOfInertiaUnits=kg*m^2  ProductsOfInertia=[0 0 0]  ProductsOfInertiaUnits=kg*m^2  BasedOnType=Density  Density=2700  DensityUnits=kg/m^3  DoExposeReferenceFrame=on  SerializedFrames=<Frames/>  GraphicType=FromGeometry  MarkerShape=Sphere  MarkerSize=10  GraphicVisPropType=AdvancedVisualProperties  GraphicDiffuseColor=[0.15 0.15 0.15]  GraphicSpecularColor=[1 1 1 1.0]  GraphicAmbientColor=[0.15 0.15 0.15 1.0]  GraphicEmissiveColor=[0. 0. 0. 1]  GraphicShininess=100  GraphicOpacity=1.0
  Point Cloud : sm_lib/Curves and Surfaces/Point Cloud  CoordinatesMatrix=Rover.new_wheel_points  CoordinatesMatrixUnits=cm  GraphicType=MarkerCloud  GraphicSphereRadius=0.5  GraphicSphereRadiusUnits=cm  GraphicVisPropType=SimpleVisualProperties  GraphicDiffuseColor=[0.07451 0.6235 1]  GraphicOpacity=1.0  GraphicSpecularColor=[0.5 0.5 0.5 1.0]  GraphicAmbientColor=[0.15 0.15 0.15 1.0]  GraphicEmissiveColor=[0.0 0.0 0.0 1.0]  GraphicShininess=75
  Rigid Transform : sm_lib/Frames and Transforms/Rigid Transform  TranslationMethod=Cartesian  TranslationStandardOffset=0  TranslationStandardOffsetUnits=m  TranslationStandardAxis=+Z  TranslationCartesianOffset=Rover.Wheel.WRJ_T  TranslationCartesianOffsetUnits=m  TranslationROffset=0  TranslationROffsetUnits=m  TranslationZOffset=0  TranslationZOffsetUnits=m  TranslationThetaOffset=0  TranslationThetaOffsetUnits=deg  RotationMethod=RotationMatrix  RotationAngleUnits=deg  RotationStandardAxis=+Z  RotationAngle=0.0  RotationArbitraryAxis=[0 0 1]  FollAlignAxisA=+X  BaseAlignAxisA=+Y  FollAlignAxisB=+Y  BaseAlignAxisB=+Z  RotationSequenceAxes=FollowerAxes  RotationSequence=XYX  RotationSequenceAngles=[0 0 0]  RotationSequenceAnglesUnits=deg  RotationMatrix=Rover.Wheel.WRJ_R  Quaternion=[1 0 0 0]
  Rigid Transform6 : sm_lib/Frames and Transforms/Rigid Transform  TranslationMethod=StandardAxis  TranslationStandardOffset=25.500/2  TranslationStandardOffsetUnits=cm  TranslationStandardAxis=+Y  TranslationCartesianOffset=[0 0 0]  TranslationCartesianOffsetUnits=cm  TranslationROffset=0  TranslationROffsetUnits=m  TranslationZOffset=0  TranslationZOffsetUnits=m  TranslationThetaOffset=0  TranslationThetaOffsetUnits=deg  RotationMethod=StandardAxis  RotationAngleUnits=deg  RotationStandardAxis=+X  RotationAngle=90  RotationArbitraryAxis=[0 0 1]  FollAlignAxisA=+X  BaseAlignAxisA=+Y  FollAlignAxisB=+Y  BaseAlignAxisB=+Z  RotationSequenceAxes=FollowerAxes  RotationSequence=XYX  RotationSequenceAngles=[0 0 0]  RotationSequenceAnglesUnits=deg  RotationMatrix=[1 0 0; 0 1 0; 0 0 1]  Quaternion=[1 0 0 0]
  WRJ : PMIOPort  Side=Right
  G : PMIOPort  Port=2  Side=Left
  connections:
  Rigid Transform6/RConn1 -- WRJ/RConn1 -- Rigid Transform/RConn1
  OuterWheel/RConn1 -- Point Cloud/LConn1 -- Rigid Transform6/LConn1
  G/RConn1 -- Point Cloud/RConn1
  InnerWheel/RConn1 -- Rigid Transform/LConn1

== system mars_rover_pose/Mars Rover Plant/Rover Plant Model/Rover /Wheels/RFWheel ==
  InnerWheel : sm_lib/Body Elements/File Solid  ExtGeomFileName=mobility_wheel_inner.stl  UnitType=Custom  ExtGeomFileUnits=cm  StepReaderType=HEX  ExportConvexHullGeometry=off  InertiaType=Custom  Mass=0  MassUnits=kg  CenterOfMass=[0 0 0]  CenterOfMassUnits=m  MomentsOfInertia=[1 1 1]*0  MomentsOfInertiaUnits=kg*m^2  ProductsOfInertia=[0 0 0]  ProductsOfInertiaUnits=kg*m^2  BasedOnType=Density  Density=1000  DensityUnits=kg/m^3  DoExposeReferenceFrame=on  SerializedFrames=<Frames/>  GraphicType=FromGeometry  MarkerShape=Sphere  MarkerSize=10  GraphicVisPropType=AdvancedVisualProperties  GraphicDiffuseColor=[1.0 1.0 1.0]  GraphicSpecularColor=[1 1 1 1.0]  GraphicAmbientColor=[0.15 0.15 0.15 1.0]  GraphicEmissiveColor=[0.1 0.1 0 1.0]  GraphicShininess=90  GraphicOpacity=1.0
  OuterWheel : sm_lib/Body Elements/File Solid  ExtGeomFileName=mobility_wheel_outer.stl  UnitType=Custom  ExtGeomFileUnits=cm  StepReaderType=HEX  ExportConvexHullGeometry=off  InertiaType=CalculateFromGeometry  Mass=1  MassUnits=kg  CenterOfMass=[0 0 0]  CenterOfMassUnits=m  MomentsOfInertia=[1 1 1]  MomentsOfInertiaUnits=kg*m^2  ProductsOfInertia=[0 0 0]  ProductsOfInertiaUnits=kg*m^2  BasedOnType=Density  Density=2700  DensityUnits=kg/m^3  DoExposeReferenceFrame=on  SerializedFrames=<Frames/>  GraphicType=FromGeometry  MarkerShape=Sphere  MarkerSize=10  GraphicVisPropType=AdvancedVisualProperties  GraphicDiffuseColor=[0.15 0.15 0.15]  GraphicSpecularColor=[1 1 1 1.0]  GraphicAmbientColor=[0.15 0.15 0.15 1.0]  GraphicEmissiveColor=[0. 0. 0. 1]  GraphicShininess=100  GraphicOpacity=1.0
  Point Cloud : sm_lib/Curves and Surfaces/Point Cloud  CoordinatesMatrix=Rover.new_wheel_points  CoordinatesMatrixUnits=cm  GraphicType=MarkerCloud  GraphicSphereRadius=0.5  GraphicSphereRadiusUnits=cm  GraphicVisPropType=SimpleVisualProperties  GraphicDiffuseColor=[0.07451 0.6235 1]  GraphicOpacity=1.0  GraphicSpecularColor=[0.5 0.5 0.5 1.0]  GraphicAmbientColor=[0.15 0.15 0.15 1.0]  GraphicEmissiveColor=[0.0 0.0 0.0 1.0]  GraphicShininess=75
  Rigid Transform : sm_lib/Frames and Transforms/Rigid Transform  TranslationMethod=Cartesian  TranslationStandardOffset=0  TranslationStandardOffsetUnits=m  TranslationStandardAxis=+Z  TranslationCartesianOffset=Rover.Wheel.WRJ_T  TranslationCartesianOffsetUnits=m  TranslationROffset=0  TranslationROffsetUnits=m  TranslationZOffset=0  TranslationZOffsetUnits=m  TranslationThetaOffset=0  TranslationThetaOffsetUnits=deg  RotationMethod=RotationMatrix  RotationAngleUnits=deg  RotationStandardAxis=+Z  RotationAngle=0.0  RotationArbitraryAxis=[0 0 1]  FollAlignAxisA=+X  BaseAlignAxisA=+Y  FollAlignAxisB=+Y  BaseAlignAxisB=+Z  RotationSequenceAxes=FollowerAxes  RotationSequence=XYX  RotationSequenceAngles=[0 0 0]  RotationSequenceAnglesUnits=deg  RotationMatrix=Rover.Wheel.WRJ_R  Quaternion=[1 0 0 0]
  Rigid Transform6 : sm_lib/Frames and Transforms/Rigid Transform  TranslationMethod=StandardAxis  TranslationStandardOffset=25.500/2  TranslationStandardOffsetUnits=cm  TranslationStandardAxis=+Y  TranslationCartesianOffset=[0 0 0]  TranslationCartesianOffsetUnits=cm  TranslationROffset=0  TranslationROffsetUnits=m  TranslationZOffset=0  TranslationZOffsetUnits=m  TranslationThetaOffset=0  TranslationThetaOffsetUnits=deg  RotationMethod=StandardAxis  RotationAngleUnits=deg  RotationStandardAxis=+X  RotationAngle=90  RotationArbitraryAxis=[0 0 1]  FollAlignAxisA=+X  BaseAlignAxisA=+Y  FollAlignAxisB=+Y  BaseAlignAxisB=+Z  RotationSequenceAxes=FollowerAxes  RotationSequence=XYX  RotationSequenceAngles=[0 0 0]  RotationSequenceAnglesUnits=deg  RotationMatrix=[1 0 0; 0 1 0; 0 0 1]  Quaternion=[1 0 0 0]
  WRJ : PMIOPort  Side=Right
  G : PMIOPort  Port=2  Side=Left
  connections:
  InnerWheel/RConn1 -- Rigid Transform/LConn1
  G/RConn1 -- Point Cloud/RConn1
  Rigid Transform6/LConn1 -- Point Cloud/LConn1 -- OuterWheel/RConn1
  Rigid Transform/RConn1 -- WRJ/RConn1 -- Rigid Transform6/RConn1

== system mars_rover_pose/Mars Rover Plant/Rover Plant Model/Rover /Wheels/RMWheel ==
  InnerWheel : sm_lib/Body Elements/File Solid  ExtGeomFileName=mobility_wheel_inner.stl  UnitType=Custom  ExtGeomFileUnits=cm  StepReaderType=HEX  ExportConvexHullGeometry=off  InertiaType=Custom  Mass=0  MassUnits=kg  CenterOfMass=[0 0 0]  CenterOfMassUnits=m  MomentsOfInertia=[1 1 1]*0  MomentsOfInertiaUnits=kg*m^2  ProductsOfInertia=[0 0 0]  ProductsOfInertiaUnits=kg*m^2  BasedOnType=Density  Density=1000  DensityUnits=kg/m^3  DoExposeReferenceFrame=on  SerializedFrames=<Frames/>  GraphicType=FromGeometry  MarkerShape=Sphere  MarkerSize=10  GraphicVisPropType=AdvancedVisualProperties  GraphicDiffuseColor=[1.0 1.0 1.0]  GraphicSpecularColor=[1 1 1 1.0]  GraphicAmbientColor=[0.15 0.15 0.15 1.0]  GraphicEmissiveColor=[0.1 0.1 0 1.0]  GraphicShininess=90  GraphicOpacity=1.0
  OuterWheel : sm_lib/Body Elements/File Solid  ExtGeomFileName=mobility_wheel_outer.stl  UnitType=Custom  ExtGeomFileUnits=cm  StepReaderType=HEX  ExportConvexHullGeometry=off  InertiaType=CalculateFromGeometry  Mass=1  MassUnits=kg  CenterOfMass=[0 0 0]  CenterOfMassUnits=m  MomentsOfInertia=[1 1 1]  MomentsOfInertiaUnits=kg*m^2  ProductsOfInertia=[0 0 0]  ProductsOfInertiaUnits=kg*m^2  BasedOnType=Density  Density=2700  DensityUnits=kg/m^3  DoExposeReferenceFrame=on  SerializedFrames=<Frames/>  GraphicType=FromGeometry  MarkerShape=Sphere  MarkerSize=10  GraphicVisPropType=AdvancedVisualProperties  GraphicDiffuseColor=[0.15 0.15 0.15]  GraphicSpecularColor=[1 1 1 1.0]  GraphicAmbientColor=[0.15 0.15 0.15 1.0]  GraphicEmissiveColor=[0. 0. 0. 1]  GraphicShininess=100  GraphicOpacity=1.0
  Point Cloud : sm_lib/Curves and Surfaces/Point Cloud  CoordinatesMatrix=Rover.new_wheel_points  CoordinatesMatrixUnits=cm  GraphicType=MarkerCloud  GraphicSphereRadius=0.5  GraphicSphereRadiusUnits=cm  GraphicVisPropType=SimpleVisualProperties  GraphicDiffuseColor=[0.07451 0.6235 1]  GraphicOpacity=1.0  GraphicSpecularColor=[0.5 0.5 0.5 1.0]  GraphicAmbientColor=[0.15 0.15 0.15 1.0]  GraphicEmissiveColor=[0.0 0.0 0.0 1.0]  GraphicShininess=75
  Rigid Transform : sm_lib/Frames and Transforms/Rigid Transform  TranslationMethod=Cartesian  TranslationStandardOffset=0  TranslationStandardOffsetUnits=m  TranslationStandardAxis=+Z  TranslationCartesianOffset=Rover.Wheel.WRJ_T  TranslationCartesianOffsetUnits=m  TranslationROffset=0  TranslationROffsetUnits=m  TranslationZOffset=0  TranslationZOffsetUnits=m  TranslationThetaOffset=0  TranslationThetaOffsetUnits=deg  RotationMethod=RotationMatrix  RotationAngleUnits=deg  RotationStandardAxis=+Z  RotationAngle=0.0  RotationArbitraryAxis=[0 0 1]  FollAlignAxisA=+X  BaseAlignAxisA=+Y  FollAlignAxisB=+Y  BaseAlignAxisB=+Z  RotationSequenceAxes=FollowerAxes  RotationSequence=XYX  RotationSequenceAngles=[0 0 0]  RotationSequenceAnglesUnits=deg  RotationMatrix=Rover.Wheel.WRJ_R  Quaternion=[1 0 0 0]
  Rigid Transform6 : sm_lib/Frames and Transforms/Rigid Transform  TranslationMethod=StandardAxis  TranslationStandardOffset=25.500/2  TranslationStandardOffsetUnits=cm  TranslationStandardAxis=+Y  TranslationCartesianOffset=[0 0 0]  TranslationCartesianOffsetUnits=cm  TranslationROffset=0  TranslationROffsetUnits=m  TranslationZOffset=0  TranslationZOffsetUnits=m  TranslationThetaOffset=0  TranslationThetaOffsetUnits=deg  RotationMethod=StandardAxis  RotationAngleUnits=deg  RotationStandardAxis=+X  RotationAngle=90  RotationArbitraryAxis=[0 0 1]  FollAlignAxisA=+X  BaseAlignAxisA=+Y  FollAlignAxisB=+Y  BaseAlignAxisB=+Z  RotationSequenceAxes=FollowerAxes  RotationSequence=XYX  RotationSequenceAngles=[0 0 0]  RotationSequenceAnglesUnits=deg  RotationMatrix=[1 0 0; 0 1 0; 0 0 1]  Quaternion=[1 0 0 0]
  WRJ : PMIOPort  Side=Right
  G : PMIOPort  Port=2  Side=Left
  connections:
  InnerWheel/RConn1 -- Rigid Transform/LConn1
  G/RConn1 -- Point Cloud/RConn1
  Rigid Transform6/LConn1 -- Point Cloud/LConn1 -- OuterWheel/RConn1
  Rigid Transform/RConn1 -- WRJ/RConn1 -- Rigid Transform6/RConn1

== system mars_rover_pose/Mars Rover Plant/Rover Plant Model/Rover /Wheels/SteeringBracketLB  ==
  File Solid5 : sm_lib/Body Elements/File Solid  ExtGeomFileName=mobility_steering_bracket.stl  UnitType=Custom  ExtGeomFileUnits=cm  StepReaderType=HEX  ExportConvexHullGeometry=off  InertiaType=CalculateFromGeometry  Mass=0  MassUnits=kg  CenterOfMass=[0 0 0]  CenterOfMassUnits=m  MomentsOfInertia=[1 1 1]*0  MomentsOfInertiaUnits=kg*m^2  ProductsOfInertia=[0 0 0]  ProductsOfInertiaUnits=kg*m^2  BasedOnType=Density  Density=1000  DensityUnits=kg/m^3  DoExposeReferenceFrame=on  SerializedFrames=<Frames/>  GraphicType=FromGeometry  MarkerShape=Sphere  MarkerSize=10  GraphicVisPropType=AdvancedVisualProperties  GraphicDiffuseColor=[0.2 0.2 0.2]  GraphicSpecularColor=[1 1 1 1.0]  GraphicAmbientColor=[0.15 0.15 0.15 1.0]  GraphicEmissiveColor=[0.0 0.0 0.0 1.0]  GraphicShininess=90  GraphicOpacity=1.0
  Reference Frame : sm_lib/Frames and Transforms/Reference Frame
  Rigid Transform : sm_lib/Frames and Transforms/Rigid Transform  TranslationMethod=Cartesian  TranslationStandardOffset=0  TranslationStandardOffsetUnits=m  TranslationStandardAxis=+Z  TranslationCartesianOffset=Rover.SB.SRJ_T  TranslationCartesianOffsetUnits=m  TranslationROffset=0  TranslationROffsetUnits=m  TranslationZOffset=0  TranslationZOffsetUnits=m  TranslationThetaOffset=0  TranslationThetaOffsetUnits=deg  RotationMethod=RotationMatrix  RotationAngleUnits=deg  RotationStandardAxis=+Z  RotationAngle=0.0  RotationArbitraryAxis=[0 0 1]  FollAlignAxisA=+X  BaseAlignAxisA=+Y  FollAlignAxisB=+Y  BaseAlignAxisB=+Z  RotationSequenceAxes=FollowerAxes  RotationSequence=XYX  RotationSequenceAngles=[0 0 0]  RotationSequenceAnglesUnits=deg  RotationMatrix=Rover.SB.SRJ_R  Quaternion=[1 0 0 0]
  Rigid Transform1 : sm_lib/Frames and Transforms/Rigid Transform  TranslationMethod=Cartesian  TranslationStandardOffset=0  TranslationStandardOffsetUnits=m  TranslationStandardAxis=+Z  TranslationCartesianOffset=Rover.SB.WRJ_T  TranslationCartesianOffsetUnits=m  TranslationROffset=0  TranslationROffsetUnits=m  TranslationZOffset=0  TranslationZOffsetUnits=m  TranslationThetaOffset=0  TranslationThetaOffsetUnits=deg  RotationMethod=RotationMatrix  RotationAngleUnits=deg  RotationStandardAxis=+Z  RotationAngle=0.0  RotationArbitraryAxis=[0 0 1]  FollAlignAxisA=+X  BaseAlignAxisA=+Y  FollAlignAxisB=+Y  BaseAlignAxisB=+Z  RotationSequenceAxes=FollowerAxes  RotationSequence=XYX  RotationSequenceAngles=[0 0 0]  RotationSequenceAnglesUnits=deg  RotationMatrix=Rover.SB.WRJ_R  Quaternion=[1 0 0 0]
  SRJ : PMIOPort  Side=Left
  WRJ : PMIOPort  Port=2  Side=Right
  connections:
  Rigid Transform/RConn1 -- SRJ/RConn1
  WRJ/RConn1 -- Rigid Transform1/RConn1
  Reference Frame/RConn1 -- Rigid Transform1/LConn1 -- Rigid Transform/LConn1 -- File Solid5/RConn1
